simulink model "w1prob1"  (R2020a)
settings: Solver=VariableStepAuto  StartTime=0.0  StopTime=10.0  RelTol=1e-3
PostLoadFcn:
  | M1=100;
  | b = 50;
  | K1 = 50;
  | M2 = 40;
  | K12 = 75;
settings Model: Creator=Anjali123  LastModifiedBy=Anjali123

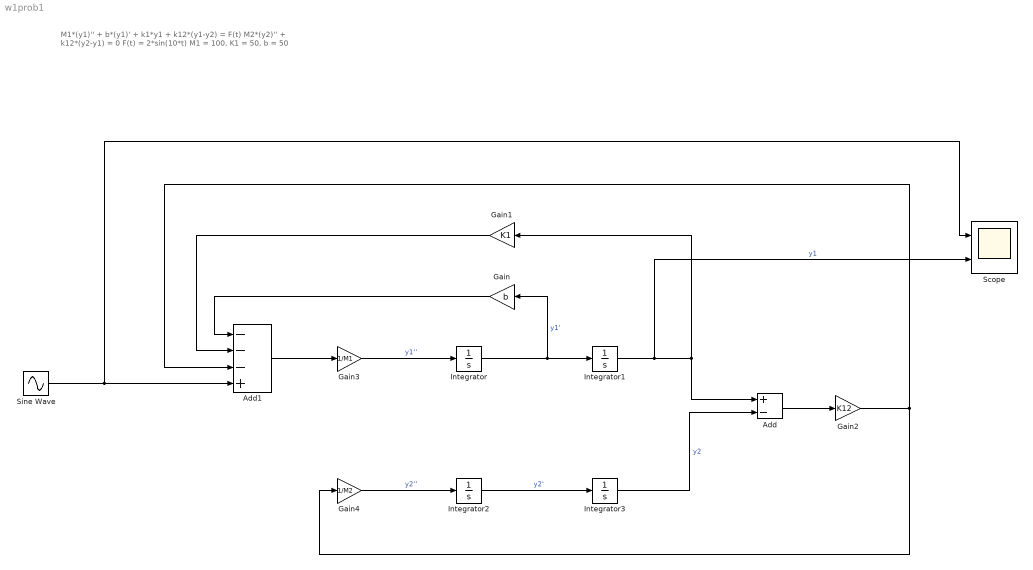
== system w1prob1 ==
  note: M1*(y1)'' + b*(y1)' + k1*y1 + k12*(y1-y2) = F(t)
      | M2*(y2)'' + k12*(y2-y1) = 0
      |
      | F(t) = 2*sin(10*t)
      | M1 = 100, K1 = 50, b = 50
  Add : Sum  Inputs=+-
  Add1 : Sum  Inputs=---+
  Gain : Gain  Gain=b
  Gain1 : Gain  Gain=K1
  Gain2 : Gain  Gain=K12
  Gain3 : Gain  Gain=1/M1
  Gain4 : Gain  Gain=1/M2
  Integrator{,1..3} (4 alike) : Integrator
  Scope : Scope  NumInputPorts=2
  Sine Wave : Sin  Amplitude=2  Frequency=10  SampleTime=0.001
  wires:
  Integrator/1 -> Gain/1, Integrator1/1  "y1'"
  Integrator1/1 -> Scope/2, Add/1, Gain1/1  "y1"
  Gain4/1 -> Integrator2/1  "y2''"
  Integrator2/1 -> Integrator3/1  "y2'"
  Integrator3/1 -> Add/2  "y2"
  Add/1 -> Gain2/1
  Gain/1 -> Add1/1
  Gain1/1 -> Add1/2
  Gain2/1 -> Gain4/1, Add1/3
  Add1/1 -> Gain3/1
  Gain3/1 -> Integrator/1  "y1''"
  Sine Wave/1 -> Scope/1, Add1/4
